simulink model "Sampling_wAliasing_AudioToolbox_a"  (R2023b)
settings: Solver=VariableStepAuto  StartTime=0.0  StopTime=inf  RelTol=1e-3  EnableMultiTasking=on
libraries: audiosources x1, dspsnks4 x1, dspvision x1, dspsrcs4 x1, dspfdesign x1, dspsigops x1
settings Model: Creator=Student  LastModifiedBy=shaanyadav
settings SolverCC: AlgebraicLoopSolver=TrustRegion
settings DataIOCC: ReturnWorkspaceOutputs=off
settings OptimizationCC: LifeSpan=inf
settings DebuggingCC: UnconnectedInputMsg=warning  UnconnectedOutputMsg=warning  UnconnectedLineMsg=warning  SFUnexpectedBacktrackingDiag=warning  SFNoUnconditionalDefaultTransitionDiag=warning  SFExecutionAtInitializationDiag=none  ArithmeticOperatorsInVariantConditions=warning
settings ModelReferenceCC: EnableRefExpFcnMdlSchedulingChecks=on
settings SFSimCC: SimUseLocalCustomCode=off  CustomCodeUndefinedFunction=UseInterfaceOnly
settings RTWCC: RTWUseLocalCustomCode=off
settings CodeAppCC: StateflowObjectComments=on
settings GRTTargetCC: TargetLangStandard=C89/C90 (ANSI)
settings ConfigComp: CovMetricSettings=dw  CovSaveCumulativeToWorkspaceVar=on  CovSaveSingleToWorkspaceVar=on  CovExternalEMLEnable=off

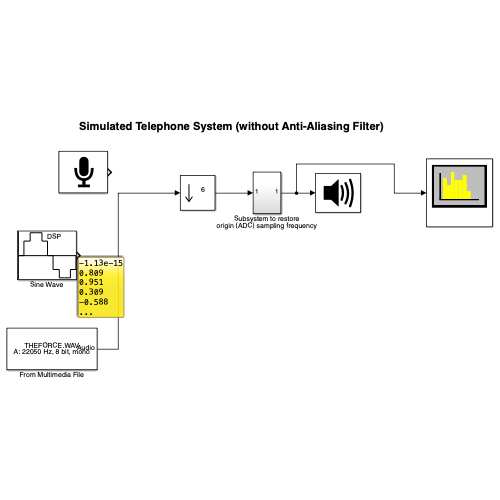
[thumbnail: Simulink's stored preview of the top-level diagram]
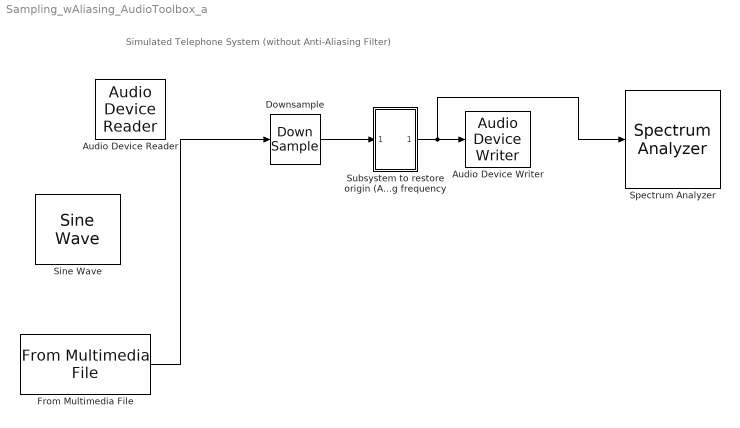
== system Sampling_wAliasing_AudioToolbox_a ==
  note: Simulated Telephone System (without Anti-Aliasing Filter)
  Audio Device Reader : audiosources/Audio Device Reader  Driver=CoreAudio  Device=Default  SampleRate=48000  NumChannels=1  SamplesPerFrame=1200  BitDepth=16-bit integer  NumBuffers=10  DefaultInputChannelMapping=on  InputChannelMapping=1:2  OutputNumOverrunSamples=off  OutputDataType=double  DriverIdx=5  DeviceWarnFlag=''
  Audio Device Writer : dspsnks4/Audio Device Writer  Driver=CoreAudio  Device=Default  InheritSampleRate=on  SampleRate=44100  BitDepth=16-bit integer  BufferSize=4096  NumBuffers=10  DefaultOutputChannelMapping=on  OutputChannelMapping=1:2  OutputNumUnderrunSamples=off  DriverIdx=5  DeviceWarnFlag=''
  Downsample : DownSample  N=6
  From Multimedia File : dspvision/From Multimedia File  inputFilename=/Users/shaanyadav/Desktop/Duke Courses/ECE 280/Lab 6 - Sampling and Aliasing/THEFORCE.WAV  readRange=[1 Inf]  loop=on  numPlays=inf  outputStreams=Audio only  videoDataType=single  audioDataType=double  inheritSampleTime=on  userDefinedSampleTime=1/30  noAudioOutput=off  isIntensityVideo=off  fourcc=RGB  colorVideoFormat=Separate color signals  outputEOF=off  dataOrg=Column-major  audioFrameSize=60  computeAudioFrameSize=off  outSamplingMode=Sample based
      settings: LibrarySourceBlock=dspsrcs4/From Multimedia File
  Sine Wave : dspsrcs4/Sine Wave  Amplitude=1  Frequency=7200  Phase=0  SampleMode=Discrete  OutComplex=Real  CompMethod=Trigonometric fcn  TableSize=Speed  SampleTime=1/48000  SamplesPerFrame=1200  ResetState=Restart at time zero  OutputFrames=off  dataType=double  wordLen=16  udDataType=sfix(16)  fracBitsMode=Best precision  numFracBits=15  OutDataTypeStr=double  LastOutDataTypeStr=double
  Spectrum Analyzer : SpectrumAnalyzer  WindowPosition=[51.000000,185.000000,1122.000000,590.000000,]  Visible=on  ScopeFrameLocation=window  Method=Welch  SampleRate=48000  AxesScaling=Manual  Span=22050  StartFrequency=-11025  StopFrequency=11025  AveragingMethod=Running  YLabel=dBm  YLimits=[-221.81259313,32.99030488]  ShowGrid=off  DefaultConfigurationName=spbscopes.SpectrumAnalyzerBlockCfg
  Subsystem to restore origin (ADC) sampling frequency : Subsystem
  wires:
  Downsample/1 -> Subsystem to restore origin (ADC) sampling frequency/1(In1)
  Subsystem to restore origin (ADC) sampling frequency/1(Out1) -> Spectrum Analyzer/1, Audio Device Writer/1
  From Multimedia File/1 -> Downsample/1

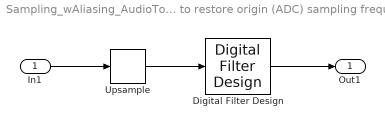
== system Sampling_wAliasing_AudioToolbox_a/Subsystem to restore origin (ADC) sampling frequency ==
  In1 : Inport
  Digital Filter Design : dspfdesign/Digital Filter Design  mwdsp_browser_bugfix_var=off
  Upsample : dspsigops/Upsample  FactorSource=Dialog parameter  N=6  Nmax=16  phase=0  InputProcessing=Columns as channels (frame based)  RateOptions=Enforce single-rate processing  ic=0  mode=Unused parameter value
  Out1 : Outport
  wires:
  In1/1 -> Upsample/1
  Upsample/1 -> Digital Filter Design/1
  Digital Filter Design/1 -> Out1/1
